simulink model "part_6"  (R2025b)
settings: Solver=VariableStepAuto  StartTime=0.0  StopTime=10.0  RelTol=1e-3
libraries: dspxfrm3 x2
settings Model: Creator=Ultor  LastModifiedBy=Ultor

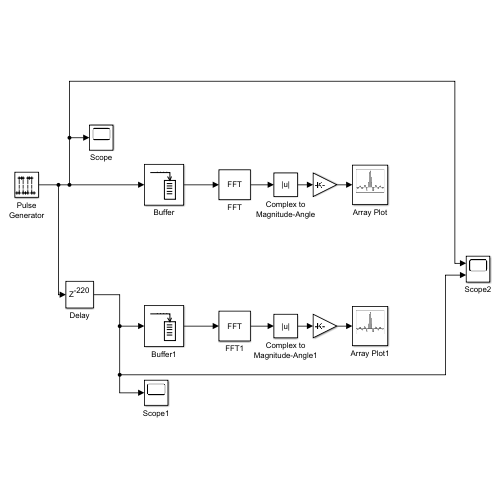
[thumbnail: Simulink's stored preview of the top-level diagram]
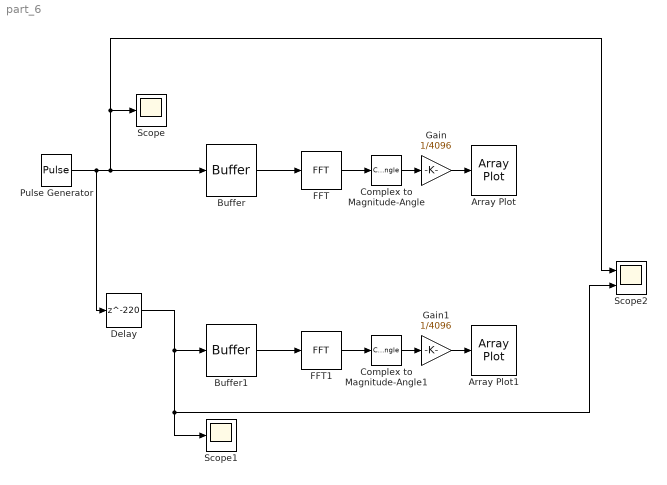
== system part_6 ==
  Array Plot : ArrayPlot  WindowPosition=[0.000000,36.000000,1920.000000,1009.000000,]  ScopeFrameLocation=window  YLimits=[-0.0132 0.1186]
  Array Plot1 : ArrayPlot  WindowPosition=[0.000000,36.000000,1920.000000,1009.000000,]  ScopeFrameLocation=window  YLimits=[-0.0132 0.1186]
  Buffer : Buffer  N=4096  OutputFrames=off
  Buffer1 : Buffer  N=4096  OutputFrames=off
  Complex to Magnitude-Angle : ComplexToMagnitudeAngle  Output=Magnitude
  Complex to Magnitude-Angle1 : ComplexToMagnitudeAngle  Output=Magnitude
  Delay : Delay  DelayLength=220
  FFT : dspxfrm3/FFT  FFTImplementation=Auto  CompMethod=Table lookup  TableOpt=NEW  TableOptActive=Speed  BitRevOrder=off  Normalize=off  InheritFFTLength=on  FFTLength=64  WrapInput=on  roundingMode=Ceiling  overflowMode=off  firstCoeffDataTypeStr=Inherit: Same word length as input  firstCoeffLastDataTypeStr=Inherit: Same word length as input  outputMin=[]  outputMax=[]
  FFT1 : dspxfrm3/FFT  FFTImplementation=Auto  CompMethod=Table lookup  TableOpt=NEW  TableOptActive=Speed  BitRevOrder=off  Normalize=off  InheritFFTLength=on  FFTLength=64  WrapInput=on  roundingMode=Ceiling  overflowMode=off  firstCoeffDataTypeStr=Inherit: Same word length as input  firstCoeffLastDataTypeStr=Inherit: Same word length as input  outputMin=[]  outputMax=[]
  Gain : Gain  Gain=1/4096
  Gain1 : Gain  Gain=1/4096
  Pulse Generator : DiscretePulseGenerator  Period=8800  PulseWidth=440  SampleTime=1/440
  Scope : Scope
      settings: ActiveDisplayYMinimum=-0.12499999999999997  ActiveDisplayYMaximum=1.125
  Scope1 : Scope
      settings: ActiveDisplayYMinimum=-0.12499999999999997  ActiveDisplayYMaximum=1.125
  Scope2 : Scope  NumInputPorts=2
      settings: ActiveDisplayYMinimum=-0.12499999999999997  ActiveDisplayYMaximum=1.125  DataLoggingVariableName=ScopeData2
  wires:
  FFT/1 -> Complex to Magnitude-Angle/1
  Complex to Magnitude-Angle/1 -> Gain/1
  Buffer/1 -> FFT/1
  Gain/1 -> Array Plot/1
  FFT1/1 -> Complex to Magnitude-Angle1/1
  Gain1/1 -> Array Plot1/1
  Pulse Generator/1 -> Delay/1, Scope/1, Scope2/1, Buffer/1
  Complex to Magnitude-Angle1/1 -> Gain1/1
  Buffer1/1 -> FFT1/1
  Delay/1 -> Buffer1/1, Scope2/2, Scope1/1
